simulink model "Laba6_1"  (R2023a)
settings: Solver=VariableStepAuto  StartTime=0.0  StopTime=10  RelTol=1e-3
values from neighbouring files (symbols this model uses):
  C_m = 1.3    [Constants.m]
  C_w = 3.15    [Constants.m]
  J_mot = 7 * 10^(-6)    (= 7e-06)    [Constants.m]
  L_a = 0.0015    [Constants.m]
  L_ov = 0.013    [Constants.m]
  R_a = 8    [Constants.m]
settings Model: Creator=manui  LastModifiedBy=manui

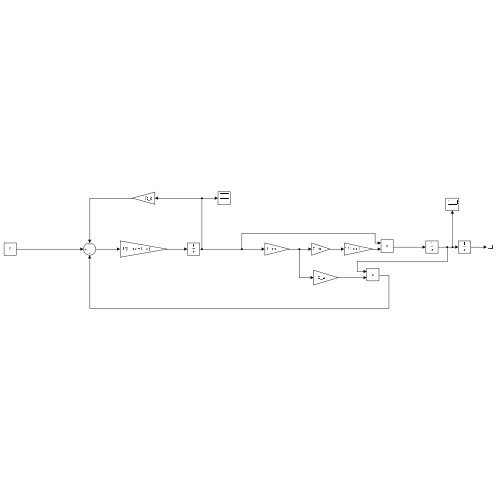
[thumbnail: Simulink's stored preview of the top-level diagram]
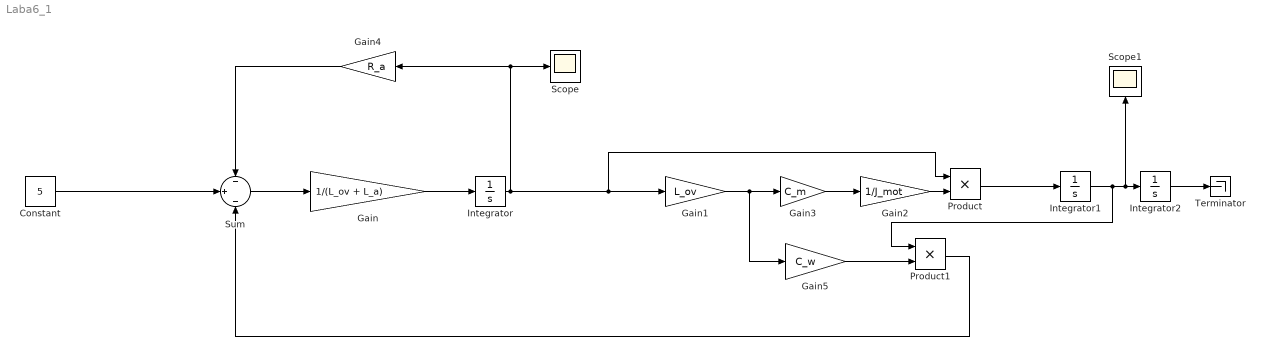
== system Laba6_1 ==
  Constant : Constant  Value=5
  Gain : Gain  Gain=1/(L_ov + L_a)
  Gain1 : Gain  Gain=L_ov
  Gain2 : Gain  Gain=1/J_mot
  Gain3 : Gain  Gain=C_m
  Gain4 : Gain  Gain=R_a
  Gain5 : Gain  Gain=C_w
  Integrator : Integrator
  Integrator1 : Integrator
  Integrator2 : Integrator
  Product : Product
  Product1 : Product
  Scope : Scope
  Scope1 : Scope
  Sum : Sum  Inputs=-|+|-
  Terminator : Terminator
  wires:
  Sum/1 -> Gain/1
  Constant/1 -> Sum/2
  Gain/1 -> Integrator/1
  Gain4/1 -> Sum/1
  Integrator/1 -> Product/1, Gain1/1, Scope/1, Gain4/1
  Gain1/1 -> Gain5/1, Gain3/1
  Gain3/1 -> Gain2/1
  Gain2/1 -> Product/2
  Product/1 -> Integrator1/1
  Integrator1/1 -> Product1/1, Scope1/1, Integrator2/1
  Integrator2/1 -> Terminator/1
  Gain5/1 -> Product1/2
  Product1/1 -> Sum/3
